simulink model "si5a_falling_ball"  (R2024a)
settings: Solver=VariableStepAuto  StartTime=0.0  StopTime=2  RelTol=1e-3
undefined symbols (not defined in the file or in its folder): g, h
libraries: simulink x1
settings Model: Creator=ocean  LastModifiedBy=ocean

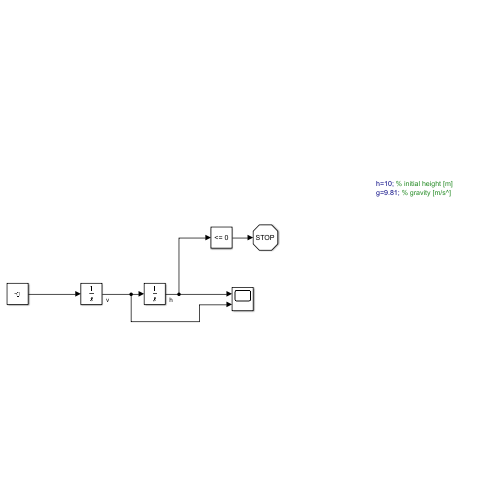
[thumbnail: Simulink's stored preview of the top-level diagram]
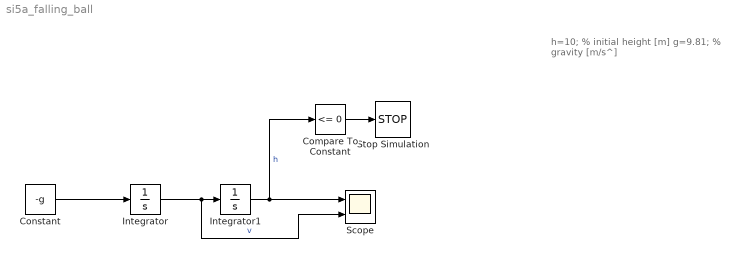
== system si5a_falling_ball ==
  note: h=10; % initial height [m]
      | g=9.81; % gravity [m/s^]
  Compare To Constant : simulink/Logic and Bit Operations/Compare To Constant  relop=<=  const=0  OutDataTypeStr=boolean
  Constant : Constant  Value=-g
  Integrator : Integrator
  Integrator1 : Integrator  InitialCondition=h
  Scope : Scope  NumInputPorts=2
  Stop Simulation : Stop
  wires:
  Constant/1 -> Integrator/1
  Integrator/1 -> Scope/2, Integrator1/1  "v"
  Integrator1/1 -> Compare To Constant/1, Scope/1  "h"
  Compare To Constant/1 -> Stop Simulation/1
